simulink model "discrete_general_system"  (R2018a)
settings: Solver=FixedStepAuto  StartTime=0.0  StopTime=3.0  FixedStep=Ti  RelTol=1e-3
undefined symbols (not defined in the file): Ad, Bd, current_correction_start, h, Ld, opt_constant_reference, opt_equilibrium_controller, opt_pwm, opt_pwm_current_controller, opt_theorem, opt_update_equilibrium, P, pwm_limit_lower, pwm_limit_upper, pwm_period, pwm_pid_kd, pwm_pid_ki, pwm_pid_kp, pwm_pid_vc_ci, pwm_pid_vc_cp, pwm_pid_vc_vi, pwm_pid_vc_vp, pwm_sample_time, Q, R, reference_controller_initial, reference_pid_ki, reference_pid_kp, Ro, sys, tau, Ts, ts, Vo, Vs, x0, xe
libraries: simulink x6, pePwmGenerator x2
settings Model: Creator=julio  LastModifiedBy=Julio-LEPO

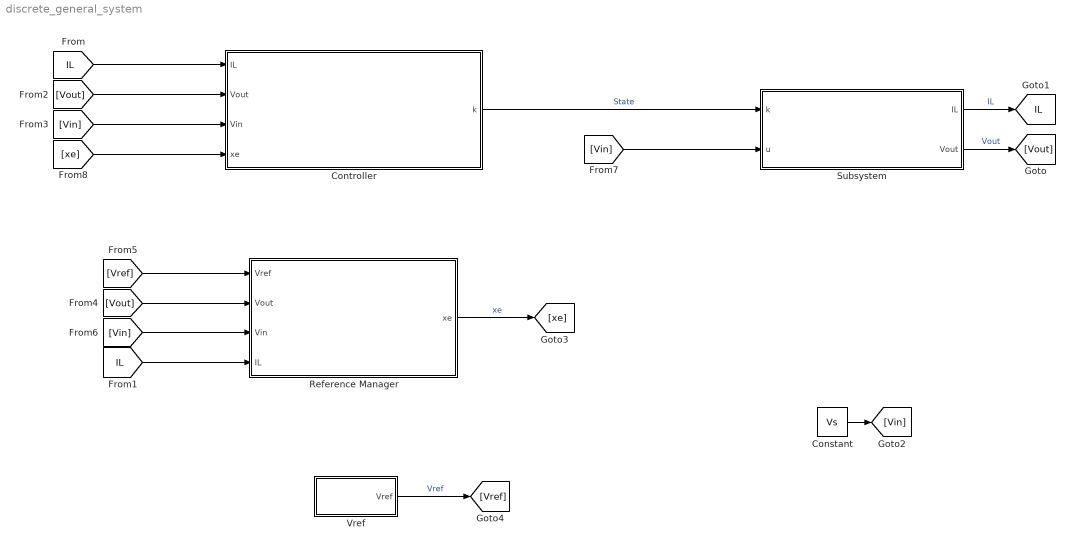
== system discrete_general_system ==
  Constant : Constant  Value=Vs
  Controller : Subsystem
  Reference Manager : Subsystem
  Subsystem : Subsystem
  Vref : Subsystem
  tag scope: IL=global
  wires:
  [Vin] -> Subsystem/2(u)
  Subsystem/1("IL ") -> [IL]  "IL"
  Subsystem/2(Vout) -> [Vout]  "Vout"
  Constant/1 -> [Vin]
  Controller/1(k) -> Subsystem/1(k)  "State"
  Vref/1(Vref) -> [Vref]  "Vref"
  [Vin] -> Reference Manager/3(Vin)
  [IL] -> Reference Manager/4(IL)
  [Vout] -> Reference Manager/2(Vout)
  [Vref] -> Reference Manager/1(Vref)
  Reference Manager/1(xe) -> [xe]  "xe"
  [IL] -> Controller/1(IL)
  [xe] -> Controller/4(xe)
  [Vin] -> Controller/3(Vin)
  [Vout] -> Controller/2(Vout)

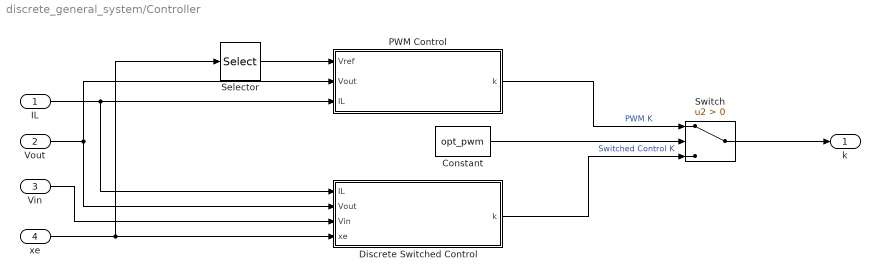
== system discrete_general_system/Controller ==
  IL : Inport
  Vout : Inport  Port=2
  Vin : Inport  Port=3
  xe : Inport  Port=4
  Constant : Constant  Value=opt_pwm
  Discrete Switched Control : Subsystem
  PWM Control : Subsystem
  Selector : Selector  InputPortWidth=2  IndexOptions=Index vector (dialog)  Indices=[2]  OutputSizes=1
  Switch : Switch  Criteria=u2 > Threshold
  k : Outport
  wires:
  IL/1 -> PWM Control/3(IL), Discrete Switched Control/1(IL)
  Vout/1 -> PWM Control/2(Vout), Discrete Switched Control/2(Vout)
  Vin/1 -> Discrete Switched Control/3(Vin)
  Switch/1 -> k/1
  Discrete Switched Control/1(k) -> Switch/3  "Switched Control K"
  Constant/1 -> Switch/2
  xe/1 -> Discrete Switched Control/4(xe), Selector/1
  Selector/1 -> PWM Control/1(Vref)
  PWM Control/1(k) -> Switch/1  "PWM K"

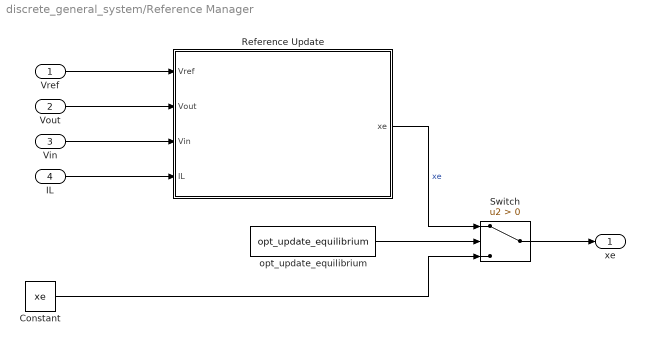
== system discrete_general_system/Reference Manager ==
  Vref : Inport
  Vout : Inport  Port=2
  Vin : Inport  Port=3
  IL : Inport  Port=4
  Constant : Constant  Value=xe
  Reference Update : Subsystem
  Switch : Switch  Criteria=u2 > Threshold
  opt_update_equilibrium : Constant  Value=opt_update_equilibrium
  xe : Outport
  wires:
  Vout/1 -> Reference Update/2(Vout)
  Vin/1 -> Reference Update/3(Vin)
  Vref/1 -> Reference Update/1(Vref)
  opt_update_equilibrium/1 -> Switch/2
  Switch/1 -> xe/1
  Reference Update/1(xe) -> Switch/1  "xe"
  Constant/1 -> Switch/3
  IL/1 -> Reference Update/4(IL)

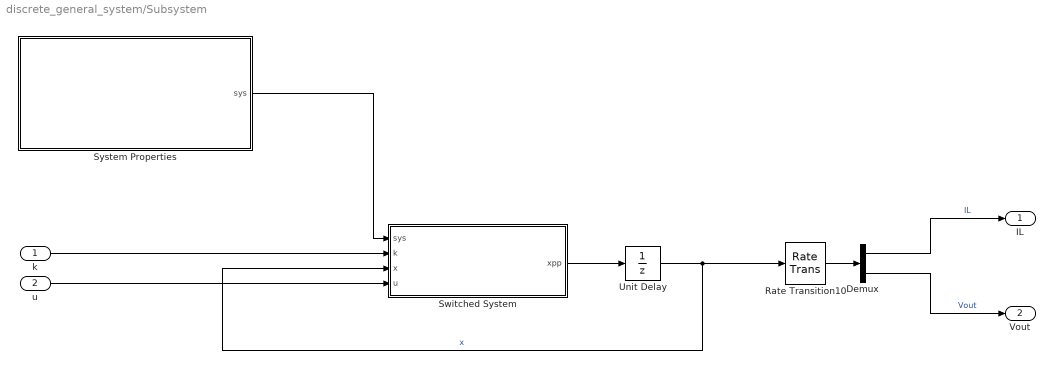
== system discrete_general_system/Subsystem ==
  k : Inport
  u : Inport  Port=2
  Demux : Demux  Outputs=2
  Rate Transition10 : RateTransition  OutPortSampleTimeOpt=Inherit  OutPortSampleTime=Ts
  Switched System : MATLAB Function  TreatAsAtomicUnit=on
  System Properties : Subsystem
  Unit Delay : UnitDelay  InitialCondition=x0  SampleTime=Ts
  "IL " : Outport
  Vout : Outport  Port=2
  wires:
  Unit Delay/1 -> Rate Transition10/1, Switched System/3(x)  "x"
  Switched System/1(xpp) -> Unit Delay/1
  k/1 -> Switched System/2(k)
  System Properties/1(sys) -> Switched System/1(sys)
  Demux/1 -> "IL "/1  "IL"
  Demux/2 -> Vout/1  "Vout"
  u/1 -> Switched System/4(u)
  Rate Transition10/1 -> Demux/1

== system discrete_general_system/Vref ==
  Constant Reference : Subsystem
  Switch1 : Switch  Criteria=u2 > Threshold
  Variable Reference : Subsystem
  opt_constant_reference : Constant  Value=opt_constant_reference
  Vref : Outport
  wires:
  opt_constant_reference/1 -> Switch1/2
  Switch1/1 -> Vref/1
  Variable Reference/1(Vref) -> Switch1/3
  Constant Reference/1(Vref) -> Switch1/1

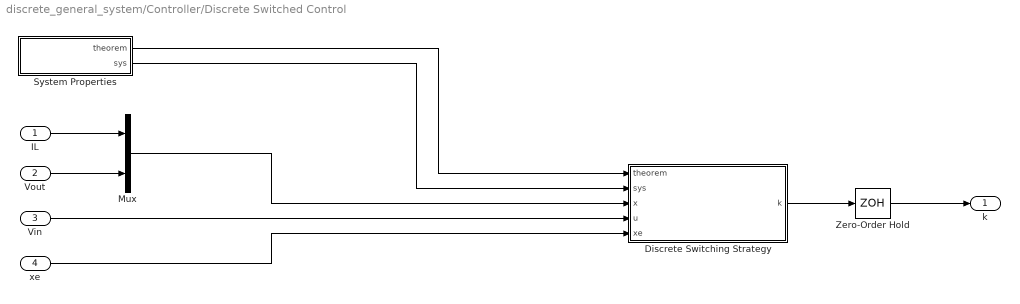
== system discrete_general_system/Controller/Discrete Switched Control ==
  IL : Inport
  Vout : Inport  Port=2
  Vin : Inport  Port=3
  xe : Inport  Port=4
  Discrete Switching Strategy : MATLAB Function  TreatAsAtomicUnit=on
  Mux : Mux  Inputs=2
  System Properties : Subsystem
  Zero-Order Hold : ZeroOrderHold  SampleTime=Ts
  k : Outport
  wires:
  Vin/1 -> Discrete Switching Strategy/4(u)
  Discrete Switching Strategy/1(k) -> Zero-Order Hold/1
  System Properties/1(theorem) -> Discrete Switching Strategy/1(theorem)
  System Properties/2(sys) -> Discrete Switching Strategy/2(sys)
  Mux/1 -> Discrete Switching Strategy/3(x)
  IL/1 -> Mux/1
  Vout/1 -> Mux/2
  xe/1 -> Discrete Switching Strategy/5(xe)
  Zero-Order Hold/1 -> k/1

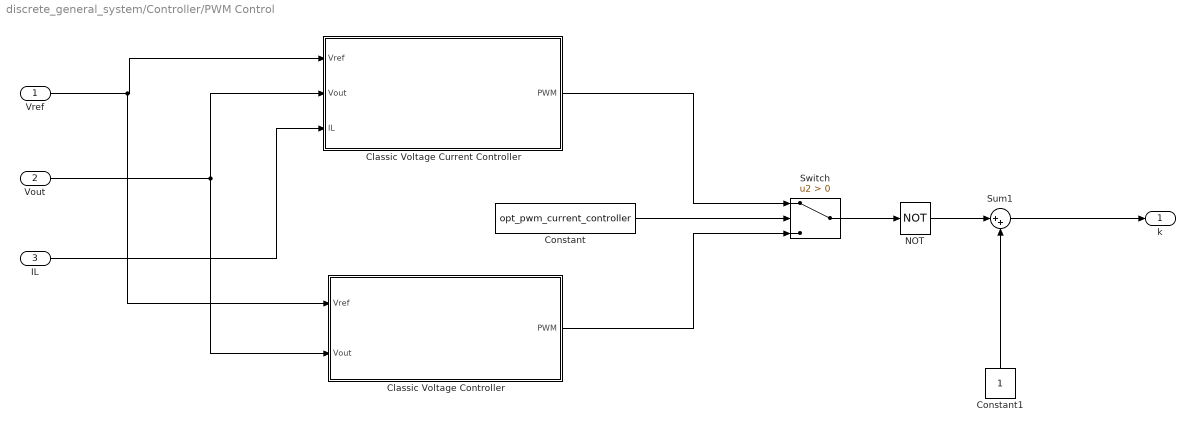
== system discrete_general_system/Controller/PWM Control ==
  Vref : Inport
  Vout : Inport  Port=2
  IL : Inport  Port=3
  Classic Voltage Controller : Subsystem
  Classic Voltage Current Controller : Subsystem
  Constant : Constant  Value=opt_pwm_current_controller
  Constant1 : Constant
  NOT : Logic  Operator=NOT  IconShape=distinctive  AllPortsSameDT=off  OutDataTypeStr=boolean
  Sum1 : Sum  Inputs=|++
  Switch : Switch  Criteria=u2 > Threshold
  k : Outport
  wires:
  Sum1/1 -> k/1
  NOT/1 -> Sum1/1
  Constant1/1 -> Sum1/2
  Vref/1 -> Classic Voltage Controller/1(Vref), Classic Voltage Current Controller/1(Vref)
  Vout/1 -> Classic Voltage Controller/2(Vout), Classic Voltage Current Controller/2(Vout)
  IL/1 -> Classic Voltage Current Controller/3(IL)
  Constant/1 -> Switch/2
  Switch/1 -> NOT/1
  Classic Voltage Controller/1(PWM) -> Switch/3
  Classic Voltage Current Controller/1(PWM) -> Switch/1

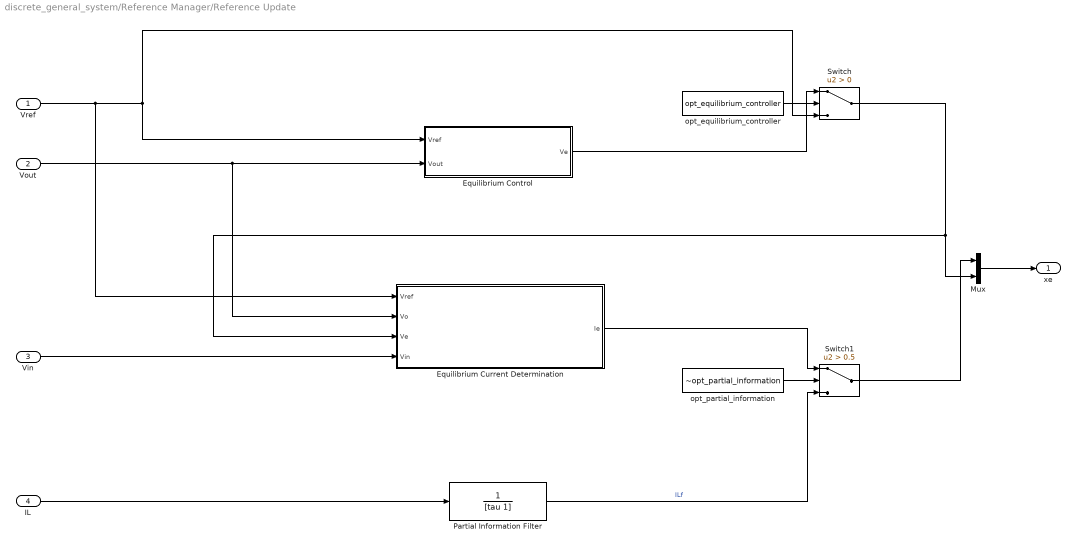
== system discrete_general_system/Reference Manager/Reference Update ==
  Vref : Inport
  Vout : Inport  Port=2
  Vin : Inport  Port=3
  IL : Inport  Port=4
  Equilibrium Control : Subsystem
  Equilibrium Current Determination : Subsystem
  Mux : Mux  Inputs=2
  Partial Information Filter : TransferFcn  Denominator=[tau 1]
  Switch : Switch  Criteria=u2 > Threshold
  Switch1 : Switch  Criteria=u2 > Threshold  Threshold=0.5
  opt_equilibrium_controller : Constant  Value=opt_equilibrium_controller
  opt_partial_information : Constant  Value=~opt_partial_information
  xe : Outport
  wires:
  Vref/1 -> Equilibrium Current Determination/1(Vref), Equilibrium Control/1(Vref), Switch/3
  Mux/1 -> xe/1
  opt_equilibrium_controller/1 -> Switch/2
  Switch/1 -> Equilibrium Current Determination/3(Ve), Mux/2
  Switch1/1 -> Mux/1
  opt_partial_information/1 -> Switch1/2
  Partial Information Filter/1 -> Switch1/3  "ILf"
  IL/1 -> Partial Information Filter/1
  Vout/1 -> Equilibrium Current Determination/2(Vo), Equilibrium Control/2(Vout)
  Equilibrium Control/1(Ve) -> Switch/1
  Vin/1 -> Equilibrium Current Determination/4(Vin)
  Equilibrium Current Determination/1(Ie) -> Switch1/1

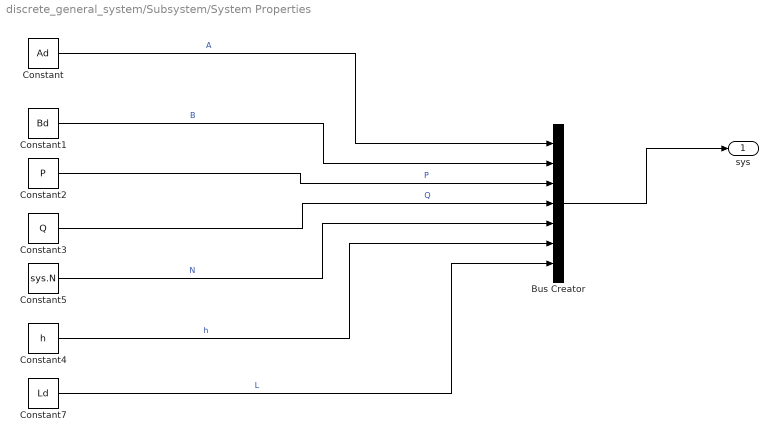
== system discrete_general_system/Subsystem/System Properties ==
  Bus Creator : BusCreator  Inputs=7  OutDataTypeStr=Bus: SystemDataBus
  Constant : Constant  Value=Ad  VectorParams1D=off
  Constant1 : Constant  Value=Bd  VectorParams1D=off
  Constant2 : Constant  Value=P  VectorParams1D=off
  Constant3 : Constant  Value=Q  VectorParams1D=off
  Constant4 : Constant  Value=h  VectorParams1D=off
  Constant5 : Constant  Value=sys.N
  Constant7 : Constant  Value=Ld  VectorParams1D=off
  sys : Outport
  wires:
  Bus Creator/1 -> sys/1
  Constant2/1 -> Bus Creator/3  "P"
  Constant1/1 -> Bus Creator/2  "B"
  Constant/1 -> Bus Creator/1  "A"
  Constant3/1 -> Bus Creator/4  "Q"
  Constant5/1 -> Bus Creator/5  "N"
  Constant4/1 -> Bus Creator/6  "h"
  Constant7/1 -> Bus Creator/7  "L"

== system discrete_general_system/Vref/Constant Reference ==
  Constant : Constant  Value=xe
  Selector : Selector  InputPortWidth=2  IndexOptions=Index vector (dialog)  Indices=[2]  OutputSizes=1
  Vref : Outport
  wires:
  Constant/1 -> Selector/1
  Selector/1 -> Vref/1

== system discrete_general_system/Vref/Variable Reference ==
  0 : Gain
  Ramp2 : simulink/Sources/Ramp  slope=Vo/ts  start=0  InitialOutput=0
  Ramp3 : simulink/Sources/Ramp  slope=Vo/ts  start=ts  InitialOutput=0
  Rate Transition10 : RateTransition  OutPortSampleTimeOpt=Inherit  OutPortSampleTime=Ts
  Sum1 : Sum  Inputs=++-
  Vdc_Ref : Step  Time=0.3  After=10  SampleTime=0
  Vref : Outport
  wires:
  Ramp2/1 -> Sum1/2
  Sum1/1 -> 0/1
  Vdc_Ref/1 -> Sum1/1
  Ramp3/1 -> Sum1/3
  0/1 -> Rate Transition10/1
  Rate Transition10/1 -> Vref/1

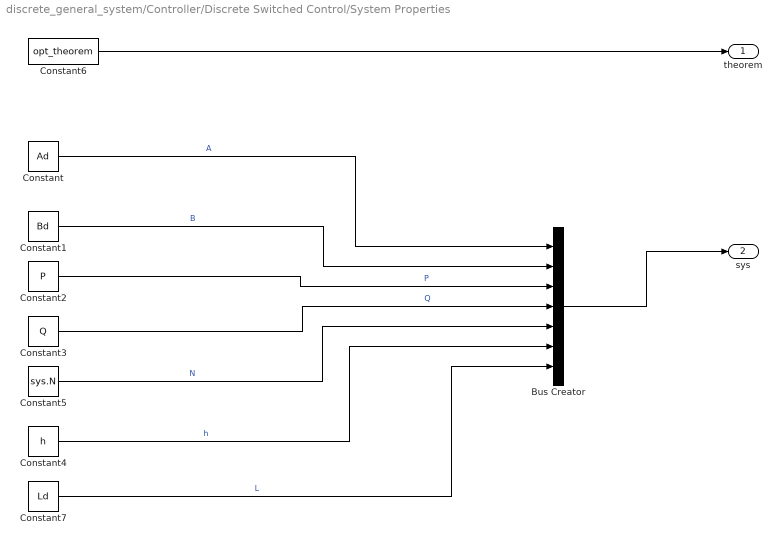
== system discrete_general_system/Controller/Discrete Switched Control/System Properties ==
  Bus Creator : BusCreator  Inputs=7  OutDataTypeStr=Bus: SystemDataBus
  Constant : Constant  Value=Ad  VectorParams1D=off
  Constant1 : Constant  Value=Bd  VectorParams1D=off
  Constant2 : Constant  Value=P  VectorParams1D=off
  Constant3 : Constant  Value=Q  VectorParams1D=off
  Constant4 : Constant  Value=h  VectorParams1D=off
  Constant5 : Constant  Value=sys.N
  Constant6 : Constant  Value=opt_theorem
  Constant7 : Constant  Value=Ld  VectorParams1D=off
  theorem : Outport
  sys : Outport  Port=2
  wires:
  Bus Creator/1 -> sys/1
  Constant2/1 -> Bus Creator/3  "P"
  Constant1/1 -> Bus Creator/2  "B"
  Constant/1 -> Bus Creator/1  "A"
  Constant3/1 -> Bus Creator/4  "Q"
  Constant5/1 -> Bus Creator/5  "N"
  Constant6/1 -> theorem/1
  Constant4/1 -> Bus Creator/6  "h"
  Constant7/1 -> Bus Creator/7  "L"

== system discrete_general_system/Controller/PWM Control/Classic Voltage Controller ==
  Vref : Inport
  Vout : Inport  Port=2
  PID Controller : simulink/Continuous/PID Controller  Controller=PI  TimeDomain=Discrete-time  SampleTime=pwm_period  IntegratorMethod=Forward Euler  FilterMethod=Forward Euler  Form=Parallel  UseFilter=on  ControllerParametersSource=internal  P=pwm_pid_kp  I=pwm_pid_ki  D=pwm_pid_kd  N=100  InitialConditionSource=internal  InitialConditionForIntegrator=0  InitialConditionForFilter=0  ExternalReset=none  LimitOutput=off  UpperSaturationLimit=inf  LowerSaturationLimit=-inf  LinearizeAsGain=on  AntiWindupMode=none  Kb=1  TrackingMode=off  Kt=1  PParamMin=[]  PParamMax=[]  IParamMin=[]  IParamMax=[]  DParamMin=[]  DParamMax=[]  NParamMin=[]  NParamMax=[]  KbParamMin=[]  KbParamMax=[]  KtParamMin=[]  KtParamMax=[]  POutMin=[]  POutMax=[]  IOutMin=[]  IOutMax=[]  DOutMin=[]  DOutMax=[]  NOutMin=[]  NOutMax=[]  KbOutMin=[]  KbOutMax=[]  KtOutMin=[]  KtOutMax=[]  IntegratorOutMin=[]  IntegratorOutMax=[]  FilterOutMin=[]  FilterOutMax=[]  SumOutMin=[]  SumOutMax=[]  SumI1OutMin=[]  SumI1OutMax=[]  SumI2OutMin=[]  SumI2OutMax=[]  SumI3OutMin=[]  SumI3OutMax=[]  SumDOutMin=[]  SumDOutMax=[]  SaturationOutMin=[]  SaturationOutMax=[]  IntegratorContinuousStateAttributes=''  IntegratorStateMustResolveToSignalObject=off  IntegratorRTWStateStorageClass=Auto  FilterContinuousStateAttributes=''  FilterStateMustResolveToSignalObject=off  FilterRTWStateStorageClass=Auto  DifferentiatorICPrevScaledInput=0  DifferentiatorOutMin=[]  DifferentiatorOutMax=[]  FilterDiffOutCoefMin=[]  FilterDiffOutCoefMax=[]  SumDenOutMin=[]  SumDenOutMax=[]  SumNumOutMin=[]  SumNumOutMax=[]  ReciprocalOutMin=[]  ReciprocalOutMax=[]  DivideOutMin=[]  DivideOutMax=[]  TunerSelectOption=Transfer Function Based (PID Tuner App)
  PWM Generator : pePwmGenerator/PWM Generator  CarrCount=Up  Tper=pwm_period  Ts=pwm_sample_time
  Saturation : Saturate  UpperLimit=pwm_limit_upper  LowerLimit=pwm_limit_lower
  Sum : Sum  Inputs=|+-
  PWM : Outport
  wires:
  Saturation/1 -> PWM Generator/1  "PWM Duty Cycle"
  PWM Generator/1 -> PWM/1
  PID Controller/1 -> Saturation/1
  Sum/1 -> PID Controller/1
  Vref/1 -> Sum/1
  Vout/1 -> Sum/2

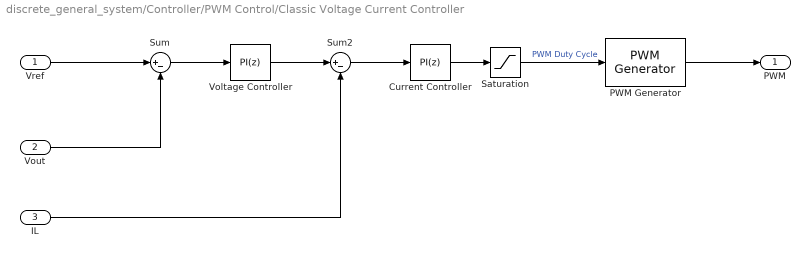
== system discrete_general_system/Controller/PWM Control/Classic Voltage Current Controller ==
  Vref : Inport
  Vout : Inport  Port=2
  IL : Inport  Port=3
  Current Controller : simulink/Continuous/PID Controller  Controller=PI  TimeDomain=Discrete-time  SampleTime=pwm_period  IntegratorMethod=Forward Euler  FilterMethod=Forward Euler  Form=Parallel  UseFilter=on  ControllerParametersSource=internal  P=pwm_pid_vc_cp  I=pwm_pid_vc_ci  D=pwm_pid_kd  N=100  InitialConditionSource=internal  InitialConditionForIntegrator=0  InitialConditionForFilter=0  ExternalReset=none  LimitOutput=off  UpperSaturationLimit=inf  LowerSaturationLimit=-inf  LinearizeAsGain=on  AntiWindupMode=none  Kb=1  TrackingMode=off  Kt=1  PParamMin=[]  PParamMax=[]  IParamMin=[]  IParamMax=[]  DParamMin=[]  DParamMax=[]  NParamMin=[]  NParamMax=[]  KbParamMin=[]  KbParamMax=[]  KtParamMin=[]  KtParamMax=[]  POutMin=[]  POutMax=[]  IOutMin=[]  IOutMax=[]  DOutMin=[]  DOutMax=[]  NOutMin=[]  NOutMax=[]  KbOutMin=[]  KbOutMax=[]  KtOutMin=[]  KtOutMax=[]  IntegratorOutMin=[]  IntegratorOutMax=[]  FilterOutMin=[]  FilterOutMax=[]  SumOutMin=[]  SumOutMax=[]  SumI1OutMin=[]  SumI1OutMax=[]  SumI2OutMin=[]  SumI2OutMax=[]  SumI3OutMin=[]  SumI3OutMax=[]  SumDOutMin=[]  SumDOutMax=[]  SaturationOutMin=[]  SaturationOutMax=[]  IntegratorContinuousStateAttributes=''  IntegratorStateMustResolveToSignalObject=off  IntegratorRTWStateStorageClass=Auto  FilterContinuousStateAttributes=''  FilterStateMustResolveToSignalObject=off  FilterRTWStateStorageClass=Auto  DifferentiatorICPrevScaledInput=0  DifferentiatorOutMin=[]  DifferentiatorOutMax=[]  FilterDiffOutCoefMin=[]  FilterDiffOutCoefMax=[]  SumDenOutMin=[]  SumDenOutMax=[]  SumNumOutMin=[]  SumNumOutMax=[]  ReciprocalOutMin=[]  ReciprocalOutMax=[]  DivideOutMin=[]  DivideOutMax=[]  TunerSelectOption=Transfer Function Based (PID Tuner App)
  PWM Generator : pePwmGenerator/PWM Generator  CarrCount=Up  Tper=pwm_period  Ts=pwm_sample_time
  Saturation : Saturate  UpperLimit=pwm_limit_upper  LowerLimit=pwm_limit_lower
  Sum : Sum  Inputs=|+-
  Sum2 : Sum  Inputs=|+-
  Voltage Controller : simulink/Continuous/PID Controller  Controller=PI  TimeDomain=Discrete-time  SampleTime=pwm_period  IntegratorMethod=Forward Euler  FilterMethod=Forward Euler  Form=Parallel  UseFilter=on  ControllerParametersSource=internal  P=pwm_pid_vc_vp  I=pwm_pid_vc_vi  D=0  N=100  InitialConditionSource=internal  InitialConditionForIntegrator=0  InitialConditionForFilter=0  ExternalReset=none  LimitOutput=off  UpperSaturationLimit=inf  LowerSaturationLimit=-inf  LinearizeAsGain=on  AntiWindupMode=none  Kb=1  TrackingMode=off  Kt=1  PParamMin=[]  PParamMax=[]  IParamMin=[]  IParamMax=[]  DParamMin=[]  DParamMax=[]  NParamMin=[]  NParamMax=[]  KbParamMin=[]  KbParamMax=[]  KtParamMin=[]  KtParamMax=[]  POutMin=[]  POutMax=[]  IOutMin=[]  IOutMax=[]  DOutMin=[]  DOutMax=[]  NOutMin=[]  NOutMax=[]  KbOutMin=[]  KbOutMax=[]  KtOutMin=[]  KtOutMax=[]  IntegratorOutMin=[]  IntegratorOutMax=[]  FilterOutMin=[]  FilterOutMax=[]  SumOutMin=[]  SumOutMax=[]  SumI1OutMin=[]  SumI1OutMax=[]  SumI2OutMin=[]  SumI2OutMax=[]  SumI3OutMin=[]  SumI3OutMax=[]  SumDOutMin=[]  SumDOutMax=[]  SaturationOutMin=[]  SaturationOutMax=[]  IntegratorContinuousStateAttributes=''  IntegratorStateMustResolveToSignalObject=off  IntegratorRTWStateStorageClass=Auto  FilterContinuousStateAttributes=''  FilterStateMustResolveToSignalObject=off  FilterRTWStateStorageClass=Auto  DifferentiatorICPrevScaledInput=0  DifferentiatorOutMin=[]  DifferentiatorOutMax=[]  FilterDiffOutCoefMin=[]  FilterDiffOutCoefMax=[]  SumDenOutMin=[]  SumDenOutMax=[]  SumNumOutMin=[]  SumNumOutMax=[]  ReciprocalOutMin=[]  ReciprocalOutMax=[]  DivideOutMin=[]  DivideOutMax=[]  TunerSelectOption=Transfer Function Based (PID Tuner App)
  PWM : Outport
  wires:
  Sum2/1 -> Current Controller/1
  Sum/1 -> Voltage Controller/1
  Vout/1 -> Sum/2
  Voltage Controller/1 -> Sum2/1
  IL/1 -> Sum2/2
  Current Controller/1 -> Saturation/1
  Vref/1 -> Sum/1
  Saturation/1 -> PWM Generator/1  "PWM Duty Cycle"
  PWM Generator/1 -> PWM/1

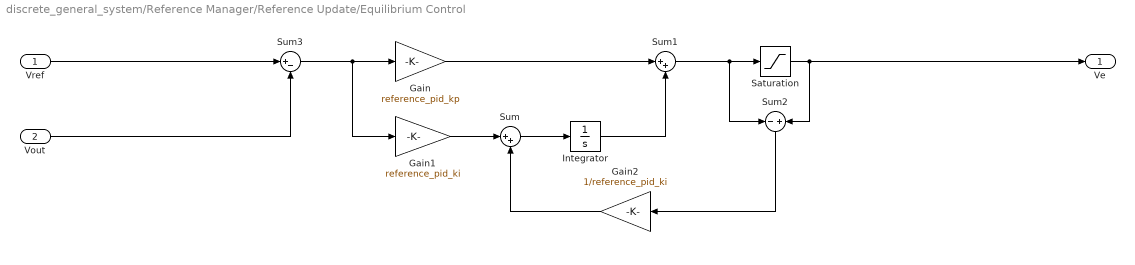
== system discrete_general_system/Reference Manager/Reference Update/Equilibrium Control ==
  Vref : Inport
  Vout : Inport  Port=2
  Gain : Gain  Gain=reference_pid_kp
  Gain1 : Gain  Gain=reference_pid_ki
  Gain2 : Gain  Gain=1/reference_pid_ki
  Integrator : Integrator  InitialCondition=reference_controller_initial
  Saturation : Saturate  UpperLimit=400  LowerLimit=0
  Sum : Sum  Inputs=|++
  Sum1 : Sum  Inputs=|++
  Sum2 : Sum  Inputs=-|+
  Sum3 : Sum  Inputs=|+-
  Ve : Outport
  wires:
  Sum1/1 -> Sum2/1, Saturation/1
  Sum/1 -> Integrator/1
  Gain1/1 -> Sum/1
  Integrator/1 -> Sum1/2
  Vout/1 -> Sum3/2
  Sum3/1 -> Gain1/1, Gain/1
  Gain/1 -> Sum1/1
  Gain2/1 -> Sum/2
  Saturation/1 -> Ve/1, Sum2/2
  Sum2/1 -> Gain2/1
  Vref/1 -> Sum3/1

== system discrete_general_system/Reference Manager/Reference Update/Equilibrium Current Determination ==
  Vref : Inport
  Vo : Inport  Port=2
  Ve : Inport  Port=3
  Vin : Inport  Port=4
  Current Correction : Subsystem
  Current Estimation : Subsystem
  Switch2 : Switch  Criteria=u2 > Threshold  Threshold=0.5
  opt_current_correction : Constant  Value=~opt_current_correction
  Ie : Outport
  wires:
  Ve/1 -> Current Estimation/1(Ve)
  Current Correction/1(Ie) -> Switch2/3
  Switch2/1 -> Ie/1
  opt_current_correction/1 -> Switch2/2
  Current Estimation/1(Ie) -> Current Correction/1(IL_e), Switch2/1
  Vref/1 -> Current Correction/2(Vref)
  Vin/1 -> Current Estimation/2(Vin)
  Vo/1 -> Current Correction/3(Vo)

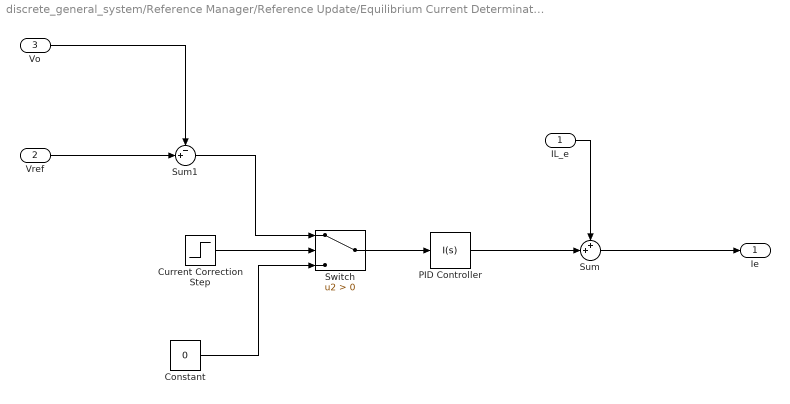
== system discrete_general_system/Reference Manager/Reference Update/Equilibrium Current Determination/Current Correction ==
  IL_e : Inport
  Vref : Inport  Port=2
  Vo : Inport  Port=3
  Constant : Constant  Value=0
  Current Correction Step : Step  Time=current_correction_start  SampleTime=0
  PID Controller : simulink/Continuous/PID Controller  Controller=I  TimeDomain=Continuous-time  SampleTime=-1  IntegratorMethod=Forward Euler  FilterMethod=Forward Euler  Form=Parallel  UseFilter=on  ControllerParametersSource=internal  P=0  I=5  D=0  N=100  InitialConditionSource=internal  InitialConditionForIntegrator=0  InitialConditionForFilter=0  ExternalReset=none  LimitOutput=off  UpperSaturationLimit=inf  LowerSaturationLimit=-inf  LinearizeAsGain=on  AntiWindupMode=none  Kb=1  TrackingMode=off  Kt=1  PParamMin=[]  PParamMax=[]  IParamMin=[]  IParamMax=[]  DParamMin=[]  DParamMax=[]  NParamMin=[]  NParamMax=[]  KbParamMin=[]  KbParamMax=[]  KtParamMin=[]  KtParamMax=[]  POutMin=[]  POutMax=[]  IOutMin=[]  IOutMax=[]  DOutMin=[]  DOutMax=[]  NOutMin=[]  NOutMax=[]  KbOutMin=[]  KbOutMax=[]  KtOutMin=[]  KtOutMax=[]  IntegratorOutMin=[]  IntegratorOutMax=[]  FilterOutMin=[]  FilterOutMax=[]  SumOutMin=[]  SumOutMax=[]  SumI1OutMin=[]  SumI1OutMax=[]  SumI2OutMin=[]  SumI2OutMax=[]  SumI3OutMin=[]  SumI3OutMax=[]  SumDOutMin=[]  SumDOutMax=[]  SaturationOutMin=[]  SaturationOutMax=[]  IntegratorContinuousStateAttributes=''  IntegratorStateMustResolveToSignalObject=off  IntegratorRTWStateStorageClass=Auto  FilterContinuousStateAttributes=''  FilterStateMustResolveToSignalObject=off  FilterRTWStateStorageClass=Auto  DifferentiatorICPrevScaledInput=0  DifferentiatorOutMin=[]  DifferentiatorOutMax=[]  FilterDiffOutCoefMin=[]  FilterDiffOutCoefMax=[]  SumDenOutMin=[]  SumDenOutMax=[]  SumNumOutMin=[]  SumNumOutMax=[]  ReciprocalOutMin=[]  ReciprocalOutMax=[]  DivideOutMin=[]  DivideOutMax=[]  TunerSelectOption=Transfer Function Based (PID Tuner App)
  Sum : Sum  Inputs=++|
  Sum1 : Sum  Inputs=-+|
  Switch : Switch  Criteria=u2 > Threshold
  Ie : Outport
  wires:
  Vo/1 -> Sum1/1
  PID Controller/1 -> Sum/2
  Sum/1 -> Ie/1
  Vref/1 -> Sum1/2
  IL_e/1 -> Sum/1
  Switch/1 -> PID Controller/1
  Current Correction Step/1 -> Switch/2
  Sum1/1 -> Switch/1
  Constant/1 -> Switch/3

== system discrete_general_system/Reference Manager/Reference Update/Equilibrium Current Determination/Current Estimation ==
  Ve : Inport
  Vin : Inport  Port=2
  Buck-Boost Equilibrium Current : MATLAB Function  TreatAsAtomicUnit=on
  Constant : Constant  Value=R
  Constant1 : Constant  Value=Ro
  Ie : Outport
  wires:
  Buck-Boost Equilibrium Current/1(I) -> Ie/1
  Constant/1 -> Buck-Boost Equilibrium Current/3(R)
  Vin/1 -> Buck-Boost Equilibrium Current/2(Vin)
  Ve/1 -> Buck-Boost Equilibrium Current/1(Ve)
  Constant1/1 -> Buck-Boost Equilibrium Current/4(Ro)

== matlab function discrete_general_system/Subsystem/Switched System ==
  data: sys input; k input; x input; u input; xpp output
function xpp = discrete_switched_system(sys, k, x, u)
    xpp = sys.A(:,:,k)*x + sys.B(:,:,k)*u;
end

== matlab function discrete_general_system/Reference Manager/Reference Update/Equilibrium Current Determination/Current Estimation/Buck-Boost Equilibrium Current ==
  data: Ve input; I output; Vin input; R input; Ro input
function I = EquilibriumCurrent(Ve, Vin, R, Ro)
    I = Vin/(2*R) - sqrt( Vin^2/(4*R^2) - Ve*(Ve+Vin)/(R*Ro) );
end

== matlab function discrete_general_system/Controller/Discrete Switched Control/Discrete Switching Strategy ==
  data: theorem input; sys input; x input; u input; k output; xe input
function k = discrete_switching_strategy(theorem, sys, x, u, xe)
    Xi = x - xe;
    sig = zeros(sys.N,1);
    
    d = sys.h'/sys.P*sys.h;
    for i=1:sys.N
        switch(theorem)
            case 1
                Xipp = sys.A(:,:,i)*Xi + sys.L(:,:,i)*u;
                sig(i) = [1 Xipp'] * [d sys.h'; sys.h sys.P] * [1; Xipp];
            case 2
                Xipp = sys.A(:,:,i)*Xi + sys.L(:,:,i)*u;
                sig(i) = [1 Xipp'] * [d sys.h'; sys.h sys.P] * [1; Xipp];
        end
    end
    [~, k] = min(sig);
end
